simulink model "gm_sampleModel1500_2_sub_sub"  (R2023a)
settings: Solver=VariableStepAuto  StartTime=0.0  StopTime=10.0  RelTol=1e-3
libraries: hdlsllib x8, simulink x3
settings Model: Creator=user1  LastModifiedBy=user1
settings OptimizationCC: BlockReduction=off  ConditionallyExecuteInputs=off
settings DebuggingCC: InheritedTsInSrcMsg=none

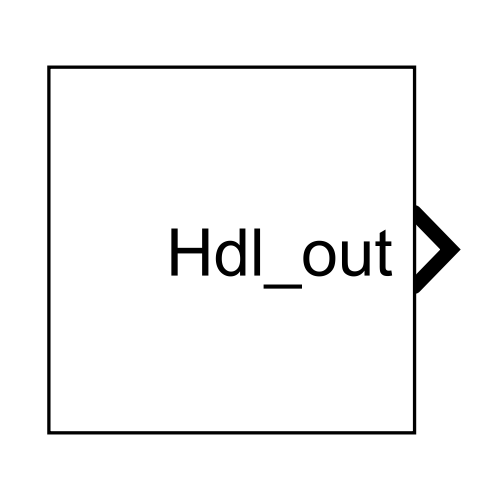
[thumbnail: Simulink's stored preview of the top-level diagram]
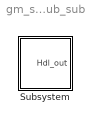
== system gm_sampleModel1500_2_sub_sub ==
  Subsystem : Subsystem

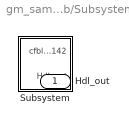
== system gm_sampleModel1500_2_sub_sub/Subsystem ==
  Subsystem : Subsystem
  Hdl_out : Outport  OutDataTypeStr=uint8

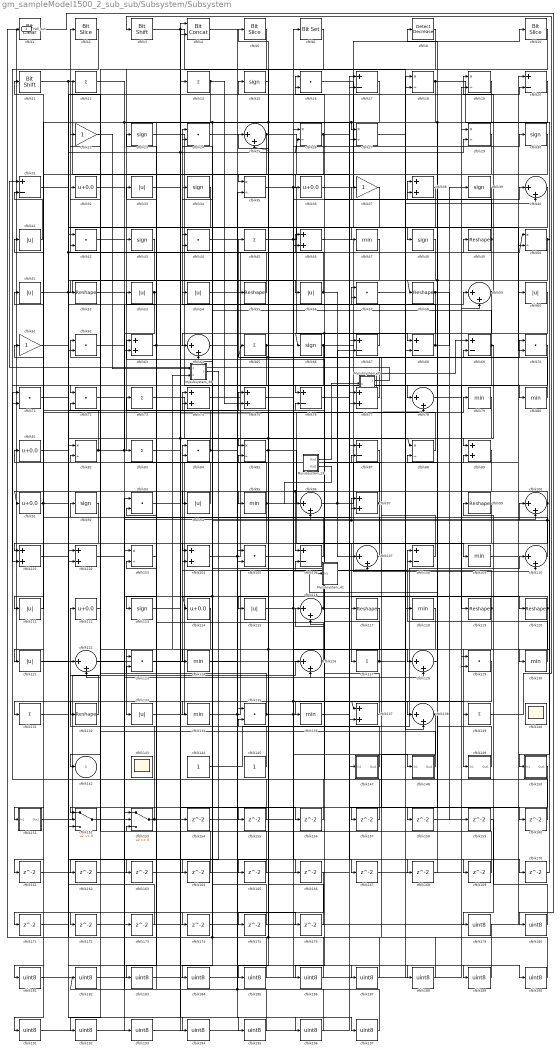
== system gm_sampleModel1500_2_sub_sub/Subsystem/Subsystem ==
  Mysubsystem_28 : Subsystem  TreatAsAtomicUnit=on  RTWFcnName=Mysubsystem_28
      settings: RTWFcnNameOpts=User specified  RTWFileNameOpts=Use function name
  Mysubsystem_35 : Subsystem  TreatAsAtomicUnit=on  RTWFcnName=Mysubsystem_35
      settings: RTWFcnNameOpts=User specified  RTWFileNameOpts=Use function name
  Mysubsystem_38 : Subsystem  TreatAsAtomicUnit=on  RTWFcnName=Mysubsystem_38
      settings: RTWFcnNameOpts=User specified  RTWFileNameOpts=Use function name
  Mysubsystem_41 : Subsystem  TreatAsAtomicUnit=on  RTWFcnName=Mysubsystem_41
      settings: RTWFcnNameOpts=User specified  RTWFileNameOpts=Use function name
  cfblk1 : simulink/Logic and Bit Operations/Bit Clear  iBit=0
      settings: LibrarySourceBlock=|
      | hdlsllib/Logic and Bit
      | Operations/Bit Clear
  cfblk10 : hdlsllib/Logic and Bit Operations/Bit Slice  lidx=7  ridx=0
  cfblk{25,40,59,64,78,96,100,107,110,116,122,126,128,138} (14 alike) : Sum  Inputs=|++  OutDataTypeStr=uint8
  cfblk{38,46,63,74..75,77,89,97,101..102,104,137} (12 alike) : Sum  OutDataTypeStr=uint8
  cfblk{18..19,26..27,29,35,50,82,85,88,103} (11 alike) : Product  Inputs=*/  OutDataTypeStr=uint8  RndMeth=Zero  SaturateOnIntegerOverflow=on
  cfblk{16,24,42,44,57,62,70..72,84,93,105,123,129,135} (15 alike) : DotProduct  OutDataTypeStr=uint8
  cfblk{17,20,31,67..69,76,87,106,108} (10 alike) : Sum  Inputs=+-  OutDataTypeStr=uint8
  cfblk{47,79..80,95,109,118,124,130,134,136} (10 alike) : MinMax  OutDataTypeStr=uint8
  cfblk11 : hdlsllib/Logic and Bit Operations/Bit Shift  mode=Shift Left Logical  N=0
  cfblk{33,41,51,53..54,56,60,94,111,115,121,133} (12 alike) : Abs  OutDataTypeStr=uint8  SaturateOnIntegerOverflow=off
  cfblk{32,36,81,91,112,114} (6 alike) : Bias  Bias=0.0  SaturateOnIntegerOverflow=off
  cfblk{15,23,30,34,39,43,48,66,92,113} (10 alike) : Signum
  cfblk{49,52,55,58,99,117,119..120,132} (9 alike) : Reshape
  cfblk{12,14,45,65,73,83,127,131,139} (9 alike) : Sum  Inputs=+  OutDataTypeStr=uint8
  cfblk140 : Scope
      settings: Floating=on
  cfblk143 : Scope
      settings: Floating=on
  cfblk144 : Constant  OutDataTypeStr=uint8  SampleTime=-1
  cfblk145 : Constant  OutDataTypeStr=uint8  SampleTime=-1
  cfblk147 : Subsystem
      settings: LibrarySourceBlock=|
      | hdlsllib/Ports &
      | Subsystems/Subsystem
  cfblk148 : Subsystem
      settings: LibrarySourceBlock=|
      | hdlsllib/Ports &
      | Subsystems/Subsystem
  cfblk149 : Subsystem
      settings: LibrarySourceBlock=|
      | hdlsllib/Ports &
      | Subsystems/Subsystem
  cfblk150 : Subsystem
      settings: LibrarySourceBlock=|
      | hdlsllib/Ports &
      | Subsystems/Subsystem
  cfblk151 : Subsystem
      settings: LibrarySourceBlock=|
      | hdlsllib/Ports &
      | Subsystems/Subsystem
  cfblk152 : Switch  OutDataTypeStr=uint8  SaturateOnIntegerOverflow=off  InputSameDT=off
  cfblk153 : Switch  OutDataTypeStr=uint8  SaturateOnIntegerOverflow=off  InputSameDT=off
  cfblk{154..176} (23 alike) : Delay  SampleTime=1
  cfblk{179..197} (19 alike) : DataTypeConversion  OutDataTypeStr=uint8  SaturateOnIntegerOverflow=off  RndMeth=Floor
  cfblk2 : hdlsllib/Logic and Bit Operations/Bit Slice  lidx=7  ridx=0
  cfblk22 : Gain  OutDataTypeStr=uint8
  cfblk3 : hdlsllib/Logic and Bit Operations/Bit Shift  mode=Shift Left Logical  N=0
  cfblk37 : Gain  OutDataTypeStr=uint8
  cfblk4 : hdlsllib/Logic and Bit Operations/Bit Concat  numInputs=2
  cfblk5 : hdlsllib/Logic and Bit Operations/Bit Slice  lidx=7  ridx=0
  cfblk6 : simulink/Logic and Bit Operations/Bit Set  iBit=0
      settings: LibrarySourceBlock=|
      | hdlsllib/Logic and Bit
      | Operations/Bit Set
  cfblk61 : Gain  OutDataTypeStr=uint8
  cfblk8 : simulink/Logic and Bit Operations/Detect Decrease  vinit=0.0  OutDataTypeStr=uint8
      settings: LibrarySourceBlock=|
      | hdlsllib/Logic and Bit
      | Operations/Detect
      | Decrease
  cfblk142 : Outport  OutDataTypeStr=uint8  VectorParamsAs1DForOutWhenUnconnected=off
  Hdl_out : Outport  Port=2  OutDataTypeStr=uint8
  wires:
  cfblk29/1 -> cfblk83/1
  cfblk35/1 -> cfblk68/1, cfblk167/1, cfblk137/1
  cfblk127/1 -> cfblk40/2, cfblk63/1
  cfblk87/1 -> cfblk186/1
  cfblk144/1 -> cfblk110/1
  cfblk4/1 -> cfblk189/1
  cfblk137/1 -> cfblk73/1
  cfblk117/1 -> cfblk133/1
  cfblk18/1 -> cfblk130/1, cfblk27/1, cfblk52/1, cfblk175/1, Mysubsystem_38/2(In2)
  cfblk108/1 -> cfblk45/1
  cfblk123/1 -> cfblk84/1
  cfblk89/1 -> cfblk91/1, cfblk106/1
  cfblk139/1 -> cfblk3/1
  cfblk145/1 -> cfblk62/1
  cfblk23/1 -> cfblk76/1
  cfblk95/1 -> cfblk142/1, cfblk64/2, cfblk79/1
  cfblk34/1 -> cfblk62/2
  cfblk133/1 -> cfblk29/1
  cfblk36/1 -> cfblk10/1
  cfblk56/1 -> cfblk107/1, cfblk2/1
  cfblk59/1 -> cfblk19/1, cfblk124/1
  cfblk10/1 -> cfblk43/1
  cfblk46/1 -> cfblk110/2
  cfblk19/1 -> cfblk151/1(In1), Mysubsystem_41/1(In1)
  cfblk81/1 -> cfblk15/1, cfblk50/1
  cfblk120/1 -> cfblk174/1, cfblk117/1
  cfblk63/1 -> cfblk183/1, cfblk77/2
  cfblk45/1 -> cfblk37/1, cfblk47/1
  cfblk109/1 -> cfblk50/2
  cfblk111/1 -> cfblk61/1
  cfblk147/1(Out1) -> cfblk112/1
  cfblk88/1 -> cfblk51/1
  cfblk118/1 -> cfblk123/1
  cfblk66/1 -> cfblk161/1, cfblk119/1
  cfblk104/1 -> cfblk57/2, cfblk70/1
  cfblk128/1 -> cfblk8/1
  cfblk83/1 -> cfblk26/2, cfblk14/1
  cfblk149/1(Out1) -> cfblk106/2
  cfblk135/1 -> cfblk32/1, cfblk40/1, cfblk148/1(In1)
  cfblk49/1 -> cfblk16/2, cfblk58/1, cfblk138/1
  cfblk110/1 -> cfblk74/2, cfblk41/1
  cfblk14/1 -> cfblk75/2, cfblk113/1
  cfblk82/1 -> cfblk11/1, cfblk57/1, cfblk85/2
  cfblk60/1 -> cfblk134/1, cfblk114/1
  cfblk151/1(Out1) -> cfblk126/1
  cfblk74/1 -> cfblk49/1
  cfblk126/1 -> Hdl_out/1, cfblk53/1
  cfblk3/1 -> cfblk78/2, cfblk68/2
  cfblk134/1 -> cfblk46/1, cfblk108/1
  cfblk11/1 -> cfblk46/2, cfblk36/1
  cfblk68/1 -> cfblk39/1, cfblk5/1
  cfblk97/1 -> cfblk76/2, cfblk127/1
  cfblk57/1 -> cfblk138/2
  cfblk92/1 -> cfblk101/1
  cfblk77/1 -> cfblk25/1, cfblk65/1
  cfblk93/1 -> cfblk195/1
  cfblk130/1 -> cfblk108/2
  cfblk65/1 -> cfblk69/2, cfblk71/2
  cfblk50/1 -> cfblk78/1, cfblk150/1(In1)
  cfblk8/1 -> cfblk132/1
  cfblk138/1 -> cfblk158/1, cfblk157/1
  cfblk52/1 -> cfblk120/1
  cfblk85/1 -> cfblk55/1, cfblk109/1
  cfblk153/1 -> cfblk72/2, cfblk26/1
  cfblk100/1 -> cfblk95/1, cfblk116/2, cfblk96/2, cfblk97/2
  cfblk33/1 -> cfblk155/1, cfblk88/1
  cfblk91/1 -> cfblk164/1, cfblk131/1
  cfblk73/1 -> cfblk147/1(In1)
  cfblk112/1 -> cfblk12/1
  cfblk53/1 -> cfblk23/1, cfblk153/2
  cfblk132/1 -> cfblk122/1
  cfblk94/1 -> cfblk81/1
  cfblk96/1 -> cfblk67/2, cfblk60/1
  cfblk5/1 -> cfblk105/2
  cfblk48/1 -> cfblk63/2
  cfblk119/1 -> cfblk104/2, cfblk149/1(In1)
  cfblk27/1 -> cfblk118/1
  cfblk115/1 -> cfblk107/2, cfblk128/1
  cfblk80/1 -> cfblk16/1
  cfblk67/1 -> cfblk24/1
  cfblk58/1 -> cfblk159/1, cfblk66/1, cfblk136/1
  cfblk99/1 -> cfblk111/1
  cfblk76/1 -> cfblk38/1
  cfblk12/1 -> cfblk166/1, cfblk27/2
  cfblk102/1 -> cfblk97/1
  cfblk16/1 -> cfblk70/2
  cfblk26/1 -> cfblk168/1, cfblk35/1
  cfblk25/1 -> cfblk67/1, cfblk121/1
  cfblk43/1 -> cfblk102/2
  cfblk116/1 -> cfblk139/1, cfblk44/1
  cfblk152/1 -> cfblk128/2
  cfblk106/1 -> cfblk22/1
  cfblk103/1 -> cfblk33/1
  cfblk37/1 -> cfblk72/1
  cfblk51/1 -> cfblk29/2, cfblk56/1
  cfblk41/1 -> cfblk31/2
  cfblk113/1 -> cfblk126/2
  cfblk2/1 -> cfblk101/2
  cfblk42/1 -> cfblk100/2
  cfblk69/1 -> cfblk24/2, cfblk137/2, cfblk89/1
  cfblk78/1 -> cfblk80/1
  cfblk20/1 -> cfblk122/2, cfblk64/1
  cfblk47/1 -> cfblk94/1
  cfblk101/1 -> cfblk20/2
  cfblk114/1 -> cfblk152/1
  cfblk75/1 -> cfblk30/1
  cfblk148/1(Out1) -> cfblk42/2
  cfblk40/1 -> cfblk104/1
  cfblk79/1 -> cfblk152/3, cfblk115/1
  cfblk105/1 -> cfblk38/2
  cfblk31/1 -> cfblk48/1
  cfblk107/1 -> cfblk92/1
  cfblk84/1 -> cfblk89/2, cfblk74/1
  cfblk6/1 -> cfblk185/1
  cfblk15/1 -> cfblk85/1
  cfblk70/1 -> cfblk152/2
  cfblk121/1 -> cfblk75/1
  cfblk55/1 -> cfblk34/1
  cfblk71/1 -> cfblk59/1
  cfblk155/1 -> cfblk42/1
  cfblk124/1 -> cfblk156/1
  cfblk156/1 -> cfblk71/1
  cfblk157/1 -> cfblk116/1
  cfblk158/1 -> cfblk59/2
  cfblk136/1 -> cfblk160/1
  cfblk160/1 -> cfblk105/1
  cfblk161/1 -> cfblk153/1
  cfblk162/1 -> cfblk35/2
  cfblk131/1 -> cfblk163/1
  cfblk163/1 -> cfblk77/1
  cfblk164/1 -> cfblk153/3
  cfblk39/1 -> cfblk165/1
  cfblk165/1 -> cfblk103/2
  cfblk167/1 -> cfblk19/2
  cfblk168/1 -> cfblk88/2
  cfblk72/1 -> cfblk169/1
  cfblk169/1 -> cfblk82/2
  cfblk24/1 -> cfblk170/1
  cfblk170/1 -> cfblk100/1
  cfblk30/1 -> cfblk171/1
  cfblk150/1(Out1) -> cfblk172/1
  cfblk172/1 -> cfblk18/2
  cfblk62/1 -> cfblk173/1
  cfblk173/1 -> cfblk102/1
  cfblk174/1 -> cfblk20/1
  cfblk175/1 -> cfblk44/2
  cfblk54/1 -> cfblk176/1
  cfblk176/1 -> cfblk135/2
  cfblk159/1 -> cfblk179/1
  cfblk179/1 -> cfblk1/1
  cfblk1/1 -> cfblk180/1
  cfblk180/1 -> cfblk99/1
  cfblk129/1 -> cfblk181/1
  cfblk181/1 -> cfblk18/1
  cfblk182/1 -> cfblk129/1
  cfblk183/1 -> cfblk129/2
  cfblk38/1 -> cfblk184/1
  cfblk184/1 -> cfblk6/1
  cfblk185/1 -> cfblk123/2, cfblk84/2
  cfblk186/1 -> cfblk103/1, cfblk54/1
  cfblk171/1 -> cfblk187/1
  cfblk187/1 -> cfblk87/1
  cfblk44/1 -> cfblk188/1
  cfblk188/1 -> cfblk87/2
  cfblk189/1 -> cfblk82/1, cfblk25/2
  cfblk64/1 -> cfblk190/1
  cfblk190/1 -> cfblk4/1
  cfblk166/1 -> cfblk191/1
  cfblk191/1 -> cfblk4/2
  cfblk17/1 -> cfblk192/1
  cfblk192/1 -> cfblk154/1
  cfblk122/1 -> cfblk193/1
  cfblk193/1 -> cfblk17/1
  cfblk32/1 -> cfblk194/1
  cfblk194/1 -> cfblk17/2
  cfblk195/1 -> cfblk135/1, cfblk182/1
  cfblk154/1 -> cfblk196/1
  cfblk196/1 -> cfblk93/1
  cfblk61/1 -> cfblk197/1
  cfblk197/1 -> cfblk93/2
  Mysubsystem_28/2(Out2) -> cfblk96/1
  Mysubsystem_28/1(Out1) -> Mysubsystem_35/1(U)
  Mysubsystem_35/1(Out1) -> cfblk31/1
  Mysubsystem_35/2(Out2) -> cfblk69/1
  cfblk22/1 -> Mysubsystem_38/1(In1)
  Mysubsystem_38/1(Out1) -> cfblk162/1

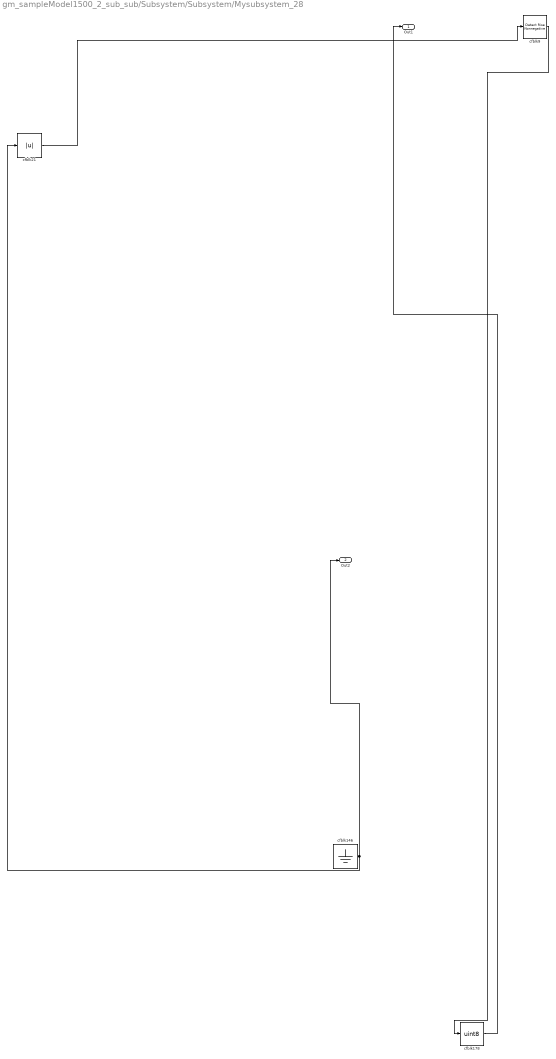
== system gm_sampleModel1500_2_sub_sub/Subsystem/Subsystem/Mysubsystem_28 ==
  cfblk146 : Ground
  cfblk178 : DataTypeConversion  OutDataTypeStr=uint8  SaturateOnIntegerOverflow=off  RndMeth=Floor
  cfblk21 : Abs  SaturateOnIntegerOverflow=off
  cfblk9 : hdlsllib/Logic and Bit Operations/Detect Rise Nonnegative  vinit=0  OutDataTypeStr=boolean
  Out1 : Outport
  Out2 : Outport  Port=2
  wires:
  cfblk21/1 -> cfblk9/1
  cfblk178/1 -> Out1/1
  cfblk146/1 -> cfblk21/1, Out2/1
  cfblk9/1 -> cfblk178/1

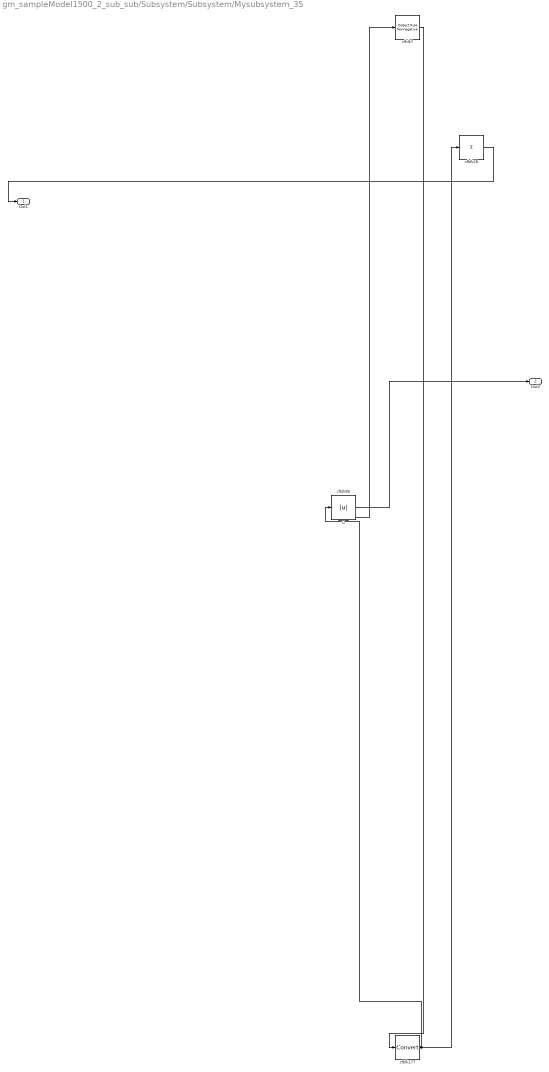
== system gm_sampleModel1500_2_sub_sub/Subsystem/Subsystem/Mysubsystem_35 ==
  U : Inport
  cfblk177 : DataTypeConversion  SaturateOnIntegerOverflow=off  RndMeth=Floor
  cfblk28 : Sum  Inputs=+
  cfblk7 : hdlsllib/Logic and Bit Operations/Detect Rise Nonnegative  vinit=0  OutDataTypeStr=boolean
  cfblk86 : Abs  SaturateOnIntegerOverflow=off
  Out1 : Outport
  Out2 : Outport  Port=2
  wires:
  cfblk86/1 -> Out2/1
  cfblk28/1 -> Out1/1
  cfblk177/1 -> cfblk86/1, cfblk28/1
  cfblk7/1 -> cfblk177/1
  U/1 -> cfblk7/1

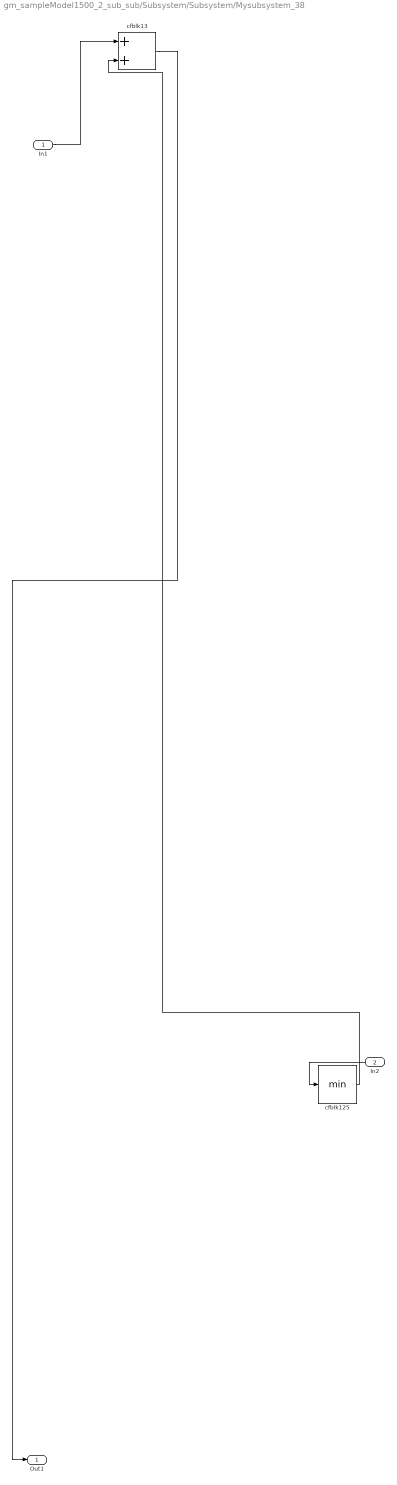
== system gm_sampleModel1500_2_sub_sub/Subsystem/Subsystem/Mysubsystem_38 ==
  In1 : Inport
  In2 : Inport  Port=2
  cfblk125 : MinMax
  cfblk13 : Sum
  Out1 : Outport
  wires:
  In2/1 -> cfblk125/1
  In1/1 -> cfblk13/1
  cfblk13/1 -> Out1/1
  cfblk125/1 -> cfblk13/2

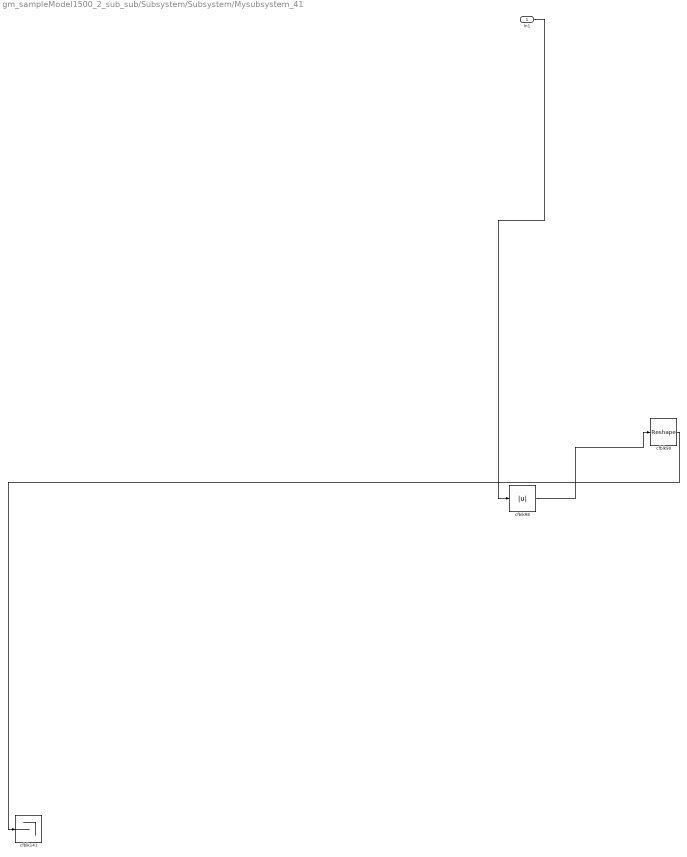
== system gm_sampleModel1500_2_sub_sub/Subsystem/Subsystem/Mysubsystem_41 ==
  In1 : Inport
  cfblk141 : Terminator
  cfblk90 : Reshape
  cfblk98 : Abs  SaturateOnIntegerOverflow=off
  wires:
  cfblk90/1 -> cfblk141/1
  In1/1 -> cfblk98/1
  cfblk98/1 -> cfblk90/1

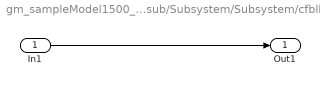
== system gm_sampleModel1500_2_sub_sub/Subsystem/Subsystem/cfblk147 ==
  In1 : Inport
  Out1 : Outport
  wires:
  In1/1 -> Out1/1

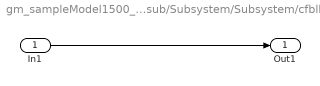
== system gm_sampleModel1500_2_sub_sub/Subsystem/Subsystem/cfblk148 ==
  In1 : Inport
  Out1 : Outport
  wires:
  In1/1 -> Out1/1

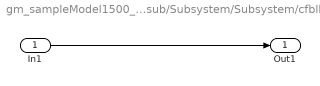
== system gm_sampleModel1500_2_sub_sub/Subsystem/Subsystem/cfblk149 ==
  In1 : Inport
  Out1 : Outport
  wires:
  In1/1 -> Out1/1

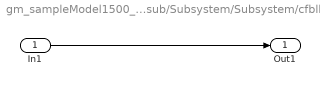
== system gm_sampleModel1500_2_sub_sub/Subsystem/Subsystem/cfblk150 ==
  In1 : Inport
  Out1 : Outport
  wires:
  In1/1 -> Out1/1

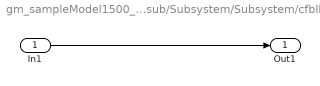
== system gm_sampleModel1500_2_sub_sub/Subsystem/Subsystem/cfblk151 ==
  In1 : Inport
  Out1 : Outport
  wires:
  In1/1 -> Out1/1
